simulink model "AWD_Test_VLC_ABS_Combined_FUZZY"  (Simulink 7.7)
settings: Solver=ode3  StartTime=0.0  StopTime=8  FixedStep=0.0001  RelTol=1e-3
undefined symbols (not defined in the file): Bx, By, Cx, Cy, Dx, Dy, Ex, Ey, g, GRR, GRR_E, hg, Jw, Jz, Lf, Lr, Lw, m, r0, Rw, rx1, rx2, ry1, ry2, T_Avail, Vx0, Vy0, wRL0
libraries: fuzblock x8, simulink x6
settings Model: Creator=ETLAB  LastModifiedBy=Kenny Schmutz
settings SolverCC: AlgebraicLoopSolver=LineSearch
settings DebuggingCC: InheritedTsInSrcMsg=none  FcnCallInpInsideContextMsg=Enable All

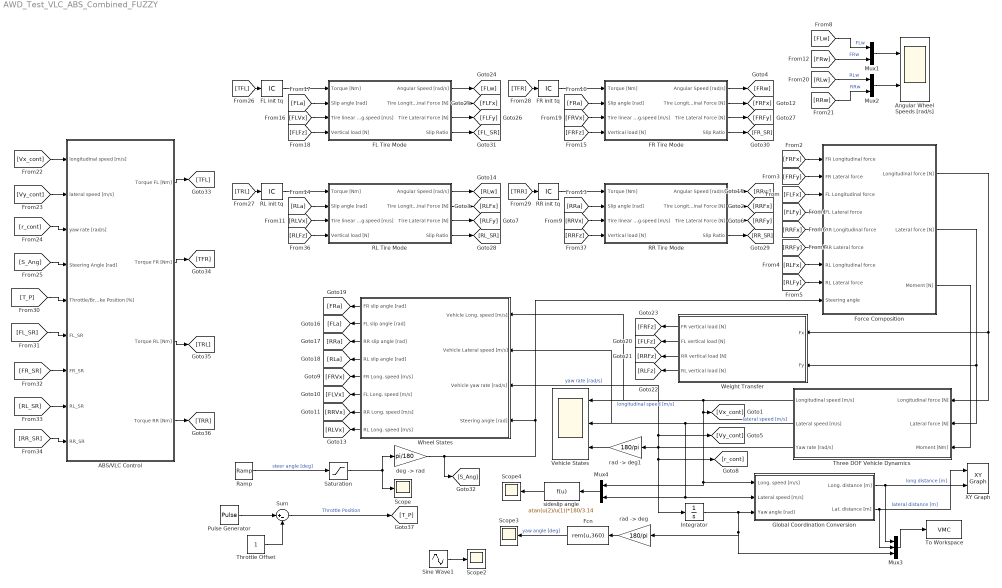
== system AWD_Test_VLC_ABS_Combined_FUZZY ==
  ABS/VLC Control : Subsystem
  Angular Wheel Speeds [rad/s] : Scope  NumInputPorts=2
      settings: YMin=-110~-110  YMax=30~30  SaveName=ScopeData7
  FL Tire Mode : Subsystem
      mask Display:
      | image(imread('Tire.bmp'),'center')
      | port_label('input', 1, 'Torque [Nm]')
      | port_label('input', 2, 'Slip angle [rad]')
      | port_label('input', 3, 'Long. speed [m/s]')
      | port_label('input', 4, 'Vertical load [N]')
      | port_label('output', 1, 'Angular speed [rad/s]')
      | port_label('output', 2, 'Long. force [N]')
      | port_label('output', 3, 'Lateral force [N]')
      | port_label('output', 4, 'Slip Ratio')
  FL init tq : InitialCondition  Value=0
  FR Tire Mode : Subsystem
      mask Display:
      | image(imread('Tire.bmp'),'center')
      | port_label('input', 1, 'Torque [Nm]')
      | port_label('input', 2, 'Slip angle [rad]')
      | port_label('input', 3, 'Long. speed [m/s]')
      | port_label('input', 4, 'Vertical load [N]')
      | port_label('output', 1, 'Angular speed [rad/s]')
      | port_label('output', 2, 'Long. force [N]')
      | port_label('output', 3, 'Lateral force [N]')
      | port_label('output', 4, 'Slip Ratio')
  FR init tq : InitialCondition  Value=0
  Fcn : Fcn  Expr=rem(u,360)
  Force Composition : Subsystem
  Global Coordination Conversion : Subsystem
  Integrator : Integrator
  Mux1 : Mux  Inputs=2
  Mux2 : Mux  Inputs=2
  Mux3 : Mux  Inputs=3
  Mux4 : Mux  Inputs=2
  Pulse Generator : DiscretePulseGenerator  PulseType=Time based  Amplitude=2  Period=8  PulseWidth=50
  RL Tire Mode : Subsystem
      mask Display:
      | image(imread('Tire.bmp'),'center')
      | port_label('input', 1, 'Torque [Nm]')
      | port_label('input', 2, 'Slip angle [rad]')
      | port_label('input', 3, 'Long. speed [m/s]')
      | port_label('input', 4, 'Vertical load [N]')
      | port_label('output', 1, 'Angular speed [rad/s]')
      | port_label('output', 2, 'Long. force [N]')
      | port_label('output', 3, 'Lateral force [N]')
      | port_label('output', 4, 'Slip Ratio')
  RL init tq : InitialCondition  Value=0
  RR Tire Mode : Subsystem
      mask Display:
      | image(imread('Tire.bmp'),'center')
      | port_label('input', 1, 'Torque [Nm]')
      | port_label('input', 2, 'Slip angle [rad]')
      | port_label('input', 3, 'Long. speed [m/s]')
      | port_label('input', 4, 'Vertical load [N]')
      | port_label('output', 1, 'Angular speed [rad/s]')
      | port_label('output', 2, 'Long. force [N]')
      | port_label('output', 3, 'Lateral force [N]')
      | port_label('output', 4, 'Slip Ratio')
  RR init tq : InitialCondition  Value=0
  Ramp : simulink/Sources/Ramp  SystemSampleTime=-1  slope=0  start=0  X0=0
  Saturation : Saturate  UpperLimit=10  LowerLimit=-10
  Scope{,2..4} (4 alike) : Scope
      Scope settings: YMin=0.93  YMax=1
      Scope2 settings: YMin=0.525  YMax=0.825  SaveName=ScopeData3
      Scope3 settings: SaveName=ScopeData5
      Scope4 settings: YMin=1.8e-014  YMax=2.5e-014  SaveName=ScopeData20
  Sine Wave1 : Sin  Frequency=0.5  SampleTime=0
  Sum : Sum  Inputs=|+-
  Three DOF Vehicle Dynamics : Subsystem
      mask Display:
      | image(imread('Vehicle.bmp'),'center')
      | port_label('input', 1, 'Longitudinal force [N]')
      | port_label('input', 2, 'Lateral force [N]')
      | port_label('input', 3, 'Moment [Nm]')
      | port_label('output', 1, 'Longitudinal speed [m/s]')
      | port_label('output', 2, 'Lateral speed [m/s]')
      | port_label('output', 3, 'Yaw rate [rad/s]')
  Throttle Offset : Constant
  To Workspace : ToWorkspace  VariableName=VMC  SampleTime=-1  SaveFormat=Array
  Vehicle States : Scope  NumInputPorts=3
      settings: TimeRange=6  YMin=2.5~-6e-018~-2.5e-016  YMax=35~5e-019~1.5e-015  SaveName=StatesOutpus1
  Weight Transfer : Subsystem
  Wheel States : Subsystem
  XY Graph : simulink/Sinks/XY Graph  SystemSampleTime=-1  xmin=-500  xmax=500  ymin=-500  ymax=500  st=-1
  "deg -> rad" : Gain  Gain=pi/180
  "rad -> deg" : Gain  Gain=180/pi
  "rad -> deg1" : Gain  Gain=180/pi
  sideslip angle : Fcn  Expr=atan(u(2)/u(1))*180/3.14
  wires:
  RL Tire Mode/2(Tire Longitudinal Force [N]) -> [RLFx]
  RL Tire Mode/1(Angular Speed [rad/s]) -> [RLw]
  [RLVx] -> RL Tire Mode/3(Tire linear Long.speed [m/s])
  Wheel States/5(FR Long. speed [m/s]) -> [FRVx]
  Wheel States/6(FL Long. speed [m/s]) -> [FLVx]
  Wheel States/7(RR Long. speed [m/s]) -> [RRVx]
  Wheel States/8(RL Long. speed [m/s]) -> [RLVx]
  Three DOF Vehicle Dynamics/3(Yaw rate [rad/s]) -> "rad -> deg1"/1, Wheel States/3(Vehicle yaw rate [rad/s]), [Vy_cont], Integrator/1, [r_cont]  "yaw rate [rad/s]"
  Three DOF Vehicle Dynamics/2(Lateral speed [m/s]) -> Wheel States/2(Vehicle Lateral speed [m/s]), Global Coordination Conversion/2(Lateral speed [m/s]), Mux4/2, Vehicle States/2  "lateral speed [m/s]"
  Three DOF Vehicle Dynamics/1(Longitudinal speed [m/s]) -> Wheel States/1(Vehicle Long. speed [m/s]), Vehicle States/1, Global Coordination Conversion/1(Long. speed [m/s]), Mux4/1, [Vx_cont]  "longitudinal speed [m/s]"
  Wheel States/1("FR slip angle [rad] ") -> [FRa]
  Wheel States/2("FL slip angle [rad] ") -> [FLa]
  Wheel States/3("RR slip angle [rad] ") -> [RRa]
  Wheel States/4("RL slip angle [rad] ") -> [RLa]
  [RLa] -> RL Tire Mode/2(Slip angle [rad])
  Force Composition/1(Longitudinal force [N]) -> Weight Transfer/1(Fx), Three DOF Vehicle Dynamics/1(Longitudinal force [N])
  [FRFx] -> Force Composition/1(FR Longitudinal force)
  [FRFy] -> Force Composition/2(FR Lateral force)
  [FLFx] -> Force Composition/3(FL Longitudinal force)
  [FLFy] -> Force Composition/4(FL Lateral force)
  [RRFx] -> Force Composition/5(RR Longitudinal force)
  [RRFy] -> Force Composition/6(RR Lateral force)
  [RLFx] -> Force Composition/7(RL Longitudinal force)
  [RLFy] -> Force Composition/8(RL Lateral force)
  "deg -> rad"/1 -> Wheel States/4(Steering angle [rad]), Force Composition/9(Steering angle), [S_Ang]
  "rad -> deg"/1 -> Fcn/1
  Fcn/1 -> Scope3/1  "yaw angle [deg]"
  Global Coordination Conversion/1(Long. distance [m]) -> XY Graph/2, Mux3/1  "long distance [m]"
  Global Coordination Conversion/2(Lat. distance [m]) -> XY Graph/1, Mux3/2  "lateral distance [m]"
  Weight Transfer/1(FR vertical load [N]) -> [FRFz]
  Weight Transfer/2(FL vertical load [N]) -> [FLFz]
  Weight Transfer/3(RR vertical load [N]) -> [RRFz]
  Weight Transfer/4(RL vertical load [N]) -> [RLFz]
  [RLFz] -> RL Tire Mode/4(Vertical load [N])
  Force Composition/2(Lateral force [N]) -> Weight Transfer/2(Fy), Three DOF Vehicle Dynamics/2(Lateral force [N])
  Integrator/1 -> Global Coordination Conversion/3(Yaw angle [rad]), "rad -> deg"/1, Mux3/3
  RL Tire Mode/3(Tire Lateral Force [N]) -> [RLFy]
  [RRa] -> RR Tire Mode/2(Slip angle [rad])
  [RRVx] -> RR Tire Mode/3(Tire linear Long.speed [m/s])
  [RRFz] -> RR Tire Mode/4(Vertical load [N])
  RR Tire Mode/1(Angular Speed [rad/s]) -> [RRw]
  RR Tire Mode/2(Tire Longitudinal Force [N]) -> [RRFx]
  RR Tire Mode/3(Tire Lateral Force [N]) -> [RRFy]
  Force Composition/3(Moment [N]) -> Three DOF Vehicle Dynamics/3(Moment [Nm])
  "rad -> deg1"/1 -> Vehicle States/3
  Mux4/1 -> sideslip angle/1
  sideslip angle/1 -> Scope4/1
  Ramp/1 -> Saturation/1  "steer angle [deg]"
  Sine Wave1/1 -> Scope2/1
  FL Tire Mode/2(Tire Longitudinal Force [N]) -> [FLFx]
  FL Tire Mode/1(Angular Speed [rad/s]) -> [FLw]
  [FLVx] -> FL Tire Mode/3(Tire linear Long.speed [m/s])
  FL init tq/1 -> FL Tire Mode/1(Torque [Nm])
  [FLa] -> FL Tire Mode/2(Slip angle [rad])
  [FLFz] -> FL Tire Mode/4(Vertical load [N])
  FL Tire Mode/3(Tire Lateral Force [N]) -> [FLFy]
  [FRa] -> FR Tire Mode/2(Slip angle [rad])
  [FRVx] -> FR Tire Mode/3(Tire linear Long.speed [m/s])
  [FRFz] -> FR Tire Mode/4(Vertical load [N])
  FR Tire Mode/1(Angular Speed [rad/s]) -> [FRw]
  FR Tire Mode/2(Tire Longitudinal Force [N]) -> [FRFx]
  FR Tire Mode/3(Tire Lateral Force [N]) -> [FRFy]
  Saturation/1 -> "deg -> rad"/1, Scope/1
  [FLw] -> Mux1/1  "FLw"
  [FRw] -> Mux1/2  "FRw"
  [RLw] -> Mux2/1  "RLw"
  [RRw] -> Mux2/2  "RRw"
  Mux1/1 -> Angular Wheel Speeds [rad/s]/1
  Mux2/1 -> Angular Wheel Speeds [rad/s]/2
  [Vx_cont] -> ABS/VLC Control/1(longitudinal speed [m/s])
  [Vy_cont] -> ABS/VLC Control/2(lateral speed [m/s])
  [r_cont] -> ABS/VLC Control/3(yaw rate [rad/s])
  RL Tire Mode/4("Slip Ratio ") -> [RL_SR]
  RR Tire Mode/4(Slip Ratio) -> [RR_SR]
  FR Tire Mode/4(Slip Ratio) -> [FR_SR]
  FL Tire Mode/4(Slip Ratio) -> [FL_SR]
  [S_Ang] -> ABS/VLC Control/4(Steering Angle [rad])
  [TFL] -> FL init tq/1
  RL init tq/1 -> RL Tire Mode/1(Torque [Nm])
  [TRL] -> RL init tq/1
  FR init tq/1 -> FR Tire Mode/1(Torque [Nm])
  [TFR] -> FR init tq/1
  RR init tq/1 -> RR Tire Mode/1(Torque [Nm])
  [TRR] -> RR init tq/1
  Sum/1 -> [T_P]  "Throttle Position"
  [T_P] -> ABS/VLC Control/5(Throttle/Brake Position [%])
  [FL_SR] -> ABS/VLC Control/6(FL_SR)
  [FR_SR] -> ABS/VLC Control/7(FR_SR)
  [RL_SR] -> ABS/VLC Control/8(RL_SR)
  [RR_SR] -> ABS/VLC Control/9(RR_SR)
  ABS/VLC Control/1(Torque FL [Nm]) -> [TFL]
  ABS/VLC Control/2(Torque FR [Nm]) -> [TFR]
  ABS/VLC Control/3(Torque RL [Nm]) -> [TRL]
  ABS/VLC Control/4(Torque RR [Nm]) -> [TRR]
  Mux3/1 -> To Workspace/1
  Pulse Generator/1 -> Sum/1
  Throttle Offset/1 -> Sum/2

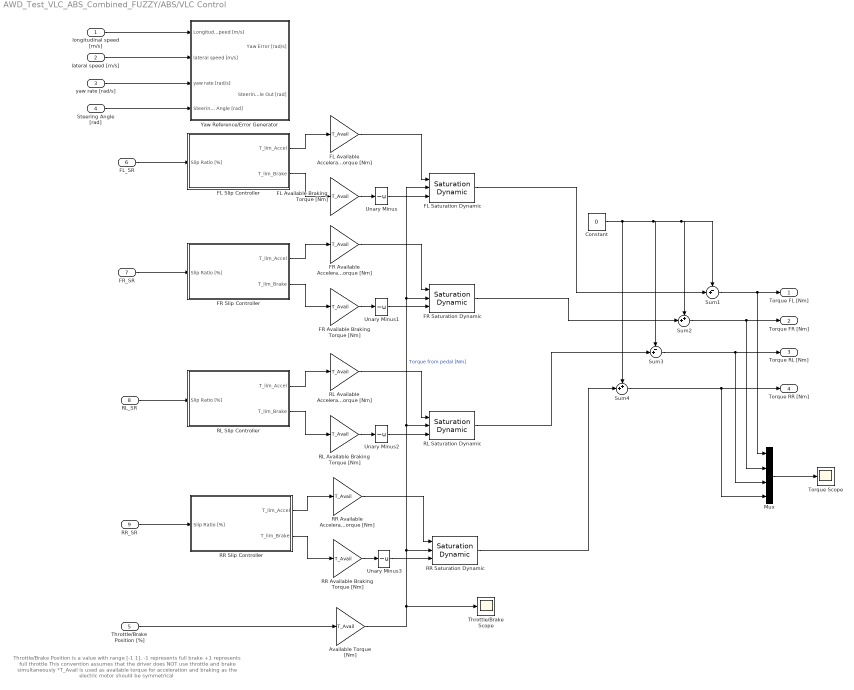
== system AWD_Test_VLC_ABS_Combined_FUZZY/ABS/VLC Control ==
  note: Throttle/Brake Position is a value with range [-1 1].
      | -1 represents full brake
      | +1 represents full throttle
      | This convention assumes that the driver does NOT use throttle and brake simultaneously
      |
      | *T_Avail is used as available torque for acceleration and braking as the electric motor should be symmetrical
  longitudinal speed [m/s] : Inport
  lateral speed [m/s] : Inport  Port=2
  yaw rate [rad/s] : Inport  Port=3
  Steering Angle [rad] : Inport  Port=4
  Throttle/Brake Position [%] : Inport  Port=5
  FL_SR : Inport  Port=6
  FR_SR : Inport  Port=7
  RL_SR : Inport  Port=8
  RR_SR : Inport  Port=9
  Available Torque [Nm] : Gain  Gain=T_Avail
  Constant : Constant  Value=0
  FL Available Acceleration Torque [Nm] : Gain  Gain=T_Avail
  FL Available Braking Torque [Nm] : Gain  Gain=T_Avail
  FL Saturation Dynamic : simulink/Discontinuities/Saturation Dynamic  SystemSampleTime=-1  OutMin=[]  OutMax=[]  OutDataTypeStr=Inherit: Same as second input  OutDataType=fixdt(1, 16)  OutScaling=2^-10  DoSatur=off
  FL Slip Controller : Subsystem
  FR Available Acceleration Torque [Nm] : Gain  Gain=T_Avail
  FR Available Braking Torque [Nm] : Gain  Gain=T_Avail
  FR Saturation Dynamic : simulink/Discontinuities/Saturation Dynamic  SystemSampleTime=-1  OutMin=[]  OutMax=[]  OutDataTypeStr=Inherit: Same as second input  OutDataType=fixdt(1, 16)  OutScaling=2^-10  DoSatur=off
  FR Slip Controller : Subsystem
  Mux : Mux
  RL Available Acceleration Torque [Nm] : Gain  Gain=T_Avail
  RL Available Braking Torque [Nm] : Gain  Gain=T_Avail
  RL Saturation Dynamic : simulink/Discontinuities/Saturation Dynamic  SystemSampleTime=-1  OutMin=[]  OutMax=[]  OutDataTypeStr=Inherit: Same as second input  OutDataType=fixdt(1, 16)  OutScaling=2^-10  DoSatur=off
  RL Slip Controller : Subsystem
  RR Available Acceleration Torque [Nm] : Gain  Gain=T_Avail
  RR Available Braking Torque [Nm] : Gain  Gain=T_Avail
  RR Saturation Dynamic : simulink/Discontinuities/Saturation Dynamic  SystemSampleTime=-1  OutMin=[]  OutMax=[]  OutDataTypeStr=Inherit: Same as second input  OutDataType=fixdt(1, 16)  OutScaling=2^-10  DoSatur=off
  RR Slip Controller : Subsystem
  Sum1 : Sum  Inputs=-+|
  Sum2 : Sum  Inputs=++|
  Sum3 : Sum  Inputs=-+|
  Sum4 : Sum  Inputs=++|
  Throttle/Brake Scope : Scope
      settings: YMin=150  YMax=150  SaveName=ScopeData9
  Torque Scope : Scope
      settings: YMin=-150  YMax=0  SaveName=ScopeData16
  Unary Minus{,1..3} (4 alike) : UnaryMinus
  Yaw Reference/Error Generator : Subsystem
  Torque FL [Nm] : Outport
  Torque FR [Nm] : Outport  Port=2
  Torque RL [Nm] : Outport  Port=3
  Torque RR [Nm] : Outport  Port=4
  wires:
  Sum1/1 -> Torque FL [Nm]/1, Mux/1
  Sum2/1 -> Torque FR [Nm]/1, Mux/2
  Sum3/1 -> Torque RL [Nm]/1, Mux/3
  Sum4/1 -> Torque RR [Nm]/1, Mux/4
  Throttle/Brake Position [%]/1 -> Available Torque [Nm]/1
  Available Torque [Nm]/1 -> RR Saturation Dynamic/2, RL Saturation Dynamic/2, FR Saturation Dynamic/2, FL Saturation Dynamic/2, Throttle/Brake Scope/1  "Torque from pedal [Nm]"
  FL_SR/1 -> FL Slip Controller/1(Slip Ratio [%])
  FL Slip Controller/1(T_lim_Accel) -> FL Available Acceleration Torque [Nm]/1
  FL Available Acceleration Torque [Nm]/1 -> FL Saturation Dynamic/1
  Unary Minus/1 -> FL Saturation Dynamic/3
  FL Saturation Dynamic/1 -> Sum1/2
  Constant/1 -> Sum4/1, Sum3/1, Sum1/1, Sum2/1
  Mux/1 -> Torque Scope/1
  FL Slip Controller/2(T_lim_Brake) -> FL Available Braking Torque [Nm]/1
  FL Available Braking Torque [Nm]/1 -> Unary Minus/1
  FR_SR/1 -> FR Slip Controller/1(Slip Ratio [%])
  FR Slip Controller/1(T_lim_Accel) -> FR Available Acceleration Torque [Nm]/1
  FR Available Acceleration Torque [Nm]/1 -> FR Saturation Dynamic/1
  Unary Minus1/1 -> FR Saturation Dynamic/3
  FR Slip Controller/2(T_lim_Brake) -> FR Available Braking Torque [Nm]/1
  FR Available Braking Torque [Nm]/1 -> Unary Minus1/1
  RL_SR/1 -> RL Slip Controller/1(Slip Ratio [%])
  RL Slip Controller/1(T_lim_Accel) -> RL Available Acceleration Torque [Nm]/1
  RL Available Acceleration Torque [Nm]/1 -> RL Saturation Dynamic/1
  Unary Minus2/1 -> RL Saturation Dynamic/3
  RL Slip Controller/2(T_lim_Brake) -> RL Available Braking Torque [Nm]/1
  RL Available Braking Torque [Nm]/1 -> Unary Minus2/1
  RR Slip Controller/1(T_lim_Accel) -> RR Available Acceleration Torque [Nm]/1
  RR Available Acceleration Torque [Nm]/1 -> RR Saturation Dynamic/1
  Unary Minus3/1 -> RR Saturation Dynamic/3
  RR Slip Controller/2(T_lim_Brake) -> RR Available Braking Torque [Nm]/1
  RR Available Braking Torque [Nm]/1 -> Unary Minus3/1
  RR_SR/1 -> RR Slip Controller/1(Slip Ratio [%])
  FR Saturation Dynamic/1 -> Sum2/2
  RL Saturation Dynamic/1 -> Sum3/2
  RR Saturation Dynamic/1 -> Sum4/2
  longitudinal speed [m/s]/1 -> Yaw Reference/Error Generator/1(Longitudinal Speed [m/s])
  lateral speed [m/s]/1 -> Yaw Reference/Error Generator/2(lateral speed [m/s])
  yaw rate [rad/s]/1 -> Yaw Reference/Error Generator/3(yaw rate [rad/s])
  Steering Angle [rad]/1 -> Yaw Reference/Error Generator/4(Steering Angle [rad])

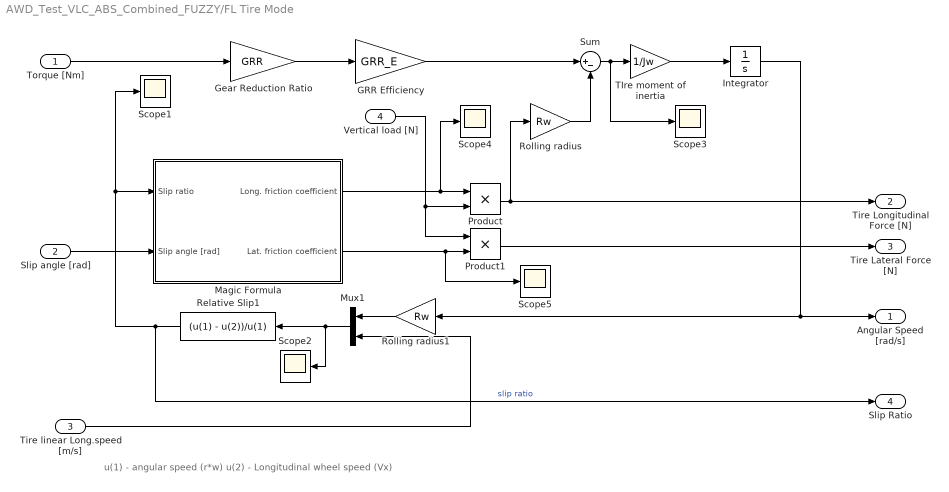
== system AWD_Test_VLC_ABS_Combined_FUZZY/FL Tire Mode ==
  note: u(1) - angular speed (r*w)
      | u(2) - Longitudinal wheel speed (Vx)
  Torque [Nm] : Inport
  Slip angle [rad] : Inport  Port=2
  Tire linear Long.speed [m/s] : Inport  Port=3
  Vertical load [N] : Inport  Port=4
  GRR Efficiency : Gain  Gain=GRR_E  SaturateOnIntegerOverflow=on  OutDataTypeStr=Inherit: Same as input  ParamDataTypeStr=Inherit: Same as input
  Gear Reduction Ratio : Gain  Gain=GRR  SaturateOnIntegerOverflow=on  OutDataTypeStr=Inherit: Same as input  ParamDataTypeStr=Inherit: Same as input
  Integrator : Integrator  InitialCondition=wRL0
  Magic Formula : Subsystem
      mask Type: Magic Formula (Combined Slip)
      mask Display:
      | image(imread('Magic formula.jpg'),'center')
      | port_label('input', 1, 'slip ratio')
      | port_label('input', 2, 'slip angle')
      | port_label('output', 1, 'Mux')
      | port_label('output', 2, 'Muy')
  Mux1 : Mux  Inputs=2
  Product : Product  RndMeth=Zero
  Product1 : Product  RndMeth=Zero
  Relative Slip1 : Fcn  Expr=(u(1) - u(2))/u(1)
  Rolling radius : Gain  Gain=Rw  SaturateOnIntegerOverflow=on  OutDataTypeStr=Inherit: Same as input  ParamDataTypeStr=Inherit: Same as input
  Rolling radius1 : Gain  Gain=Rw  SaturateOnIntegerOverflow=on  OutDataTypeStr=Inherit: Same as input  ParamDataTypeStr=Inherit: Same as input
  Scope{1..5} (5 alike) : Scope
      Scope1 settings: YMin=0.122  YMax=0.122004  SaveName=ScopeData2
      Scope2 settings: TimeRange=6  YMin=44  YMax=50.5  SaveName=ScopeData11
      Scope3 settings: YMin=5.45315  YMax=5.45315  SaveName=ScopeData14
      Scope4 settings: YMin=0.775111  YMax=0.856701  SaveName=ScopeData13
      Scope5 settings: YMin=-0.14725  YMax=-0.1463  SaveName=ScopeData15
  Sum : Sum  Inputs=|+-
  TIre moment of inertia : Gain  Gain=1/Jw  SaturateOnIntegerOverflow=on  OutDataTypeStr=Inherit: Same as input  ParamDataTypeStr=Inherit: Same as input
  Angular Speed [rad/s] : Outport
  Tire Longitudinal Force [N] : Outport  Port=2
  Tire Lateral Force [N] : Outport  Port=3
  Slip Ratio : Outport  Port=4
  wires:
  Slip angle [rad]/1 -> Magic Formula/2(Slip angle [rad])
  Relative Slip1/1 -> Magic Formula/1(Slip ratio), Scope1/1, Slip Ratio/1  "slip ratio"
  Tire linear Long.speed [m/s]/1 -> Mux1/2
  Torque [Nm]/1 -> Gear Reduction Ratio/1
  Sum/1 -> TIre moment of inertia/1, Scope3/1
  TIre moment of inertia/1 -> Integrator/1
  Integrator/1 -> Angular Speed [rad/s]/1, Rolling radius1/1
  Rolling radius/1 -> Sum/2
  Mux1/1 -> Relative Slip1/1, Scope2/1
  Rolling radius1/1 -> Mux1/1
  Magic Formula/1(Long. friction coefficient) -> Product/1, Scope4/1
  Magic Formula/2(Lat. friction coefficient) -> Product1/2, Scope5/1
  Product/1 -> Rolling radius/1, Tire Longitudinal Force [N]/1
  Vertical load [N]/1 -> Product/2, Product1/1
  Product1/1 -> Tire Lateral Force [N]/1
  Gear Reduction Ratio/1 -> GRR Efficiency/1
  GRR Efficiency/1 -> Sum/1

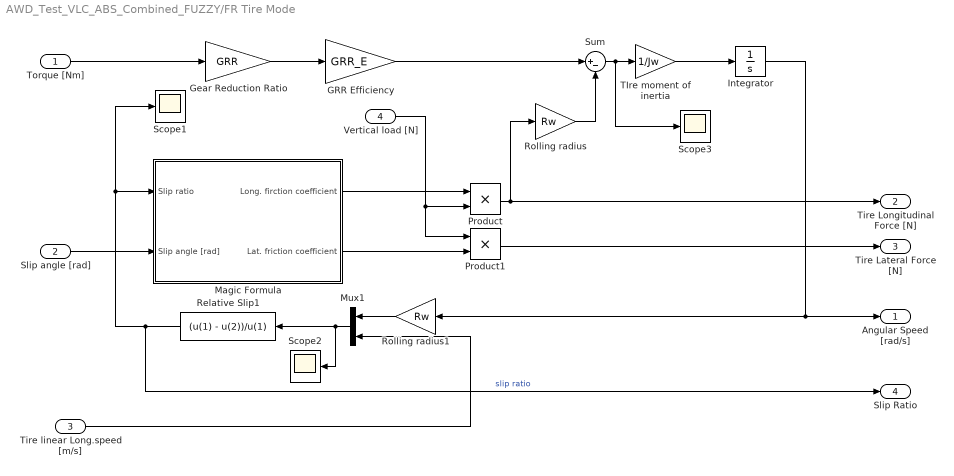
== system AWD_Test_VLC_ABS_Combined_FUZZY/FR Tire Mode ==
  Torque [Nm] : Inport
  Slip angle [rad] : Inport  Port=2
  Tire linear Long.speed [m/s] : Inport  Port=3
  Vertical load [N] : Inport  Port=4
  GRR Efficiency : Gain  Gain=GRR_E  SaturateOnIntegerOverflow=on  OutDataTypeStr=Inherit: Same as input  ParamDataTypeStr=Inherit: Same as input
  Gear Reduction Ratio : Gain  Gain=GRR  SaturateOnIntegerOverflow=on  OutDataTypeStr=Inherit: Same as input  ParamDataTypeStr=Inherit: Same as input
  Integrator : Integrator  InitialCondition=wRL0
  Magic Formula : Subsystem
      mask Type: Magic Formula (Combined Slip)
      mask Display:
      | image(imread('Magic formula.jpg'),'center')
      | port_label('input', 1, 'slip ratio')
      | port_label('input', 2, 'slip angle')
      | port_label('output', 1, 'Mux')
      | port_label('output', 2, 'Muy')
  Mux1 : Mux  Inputs=2
  Product : Product  RndMeth=Zero
  Product1 : Product  RndMeth=Zero
  Relative Slip1 : Fcn  Expr=(u(1) - u(2))/u(1)
  Rolling radius : Gain  Gain=Rw  SaturateOnIntegerOverflow=on  OutDataTypeStr=Inherit: Same as input  ParamDataTypeStr=Inherit: Same as input
  Rolling radius1 : Gain  Gain=Rw  SaturateOnIntegerOverflow=on  OutDataTypeStr=Inherit: Same as input  ParamDataTypeStr=Inherit: Same as input
  Scope1 : Scope
      settings: YMin=0.0014905  YMax=0.0014955  SaveName=ScopeData2
  Scope2 : Scope
      settings: YMin=0.001  YMax=0.013  SaveName=ScopeData11
  Scope3 : Scope
      settings: SaveName=ScopeData14
  Sum : Sum  Inputs=|+-
  TIre moment of inertia : Gain  Gain=1/Jw  SaturateOnIntegerOverflow=on  OutDataTypeStr=Inherit: Same as input  ParamDataTypeStr=Inherit: Same as input
  Angular Speed [rad/s] : Outport
  Tire Longitudinal Force [N] : Outport  Port=2
  Tire Lateral Force [N] : Outport  Port=3
  Slip Ratio : Outport  Port=4
  wires:
  Product1/1 -> Tire Lateral Force [N]/1
  Vertical load [N]/1 -> Product1/1, Product/2
  Product/1 -> Tire Longitudinal Force [N]/1, Rolling radius/1
  Magic Formula/2(Lat. friction coefficient) -> Product1/2
  Magic Formula/1(Long. firction coefficient) -> Product/1
  Rolling radius1/1 -> Mux1/1
  Mux1/1 -> Relative Slip1/1, Scope2/1
  Rolling radius/1 -> Sum/2
  Integrator/1 -> Rolling radius1/1, Angular Speed [rad/s]/1
  TIre moment of inertia/1 -> Integrator/1
  Sum/1 -> Scope3/1, TIre moment of inertia/1
  Torque [Nm]/1 -> Gear Reduction Ratio/1
  Tire linear Long.speed [m/s]/1 -> Mux1/2
  Relative Slip1/1 -> Scope1/1, Magic Formula/1(Slip ratio), Slip Ratio/1  "slip ratio"
  Slip angle [rad]/1 -> Magic Formula/2(Slip angle [rad])
  Gear Reduction Ratio/1 -> GRR Efficiency/1
  GRR Efficiency/1 -> Sum/1

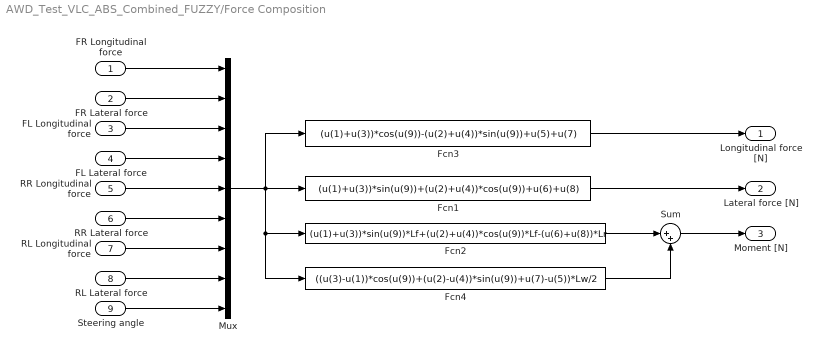
== system AWD_Test_VLC_ABS_Combined_FUZZY/Force Composition ==
  FR Longitudinal force : Inport
  FR Lateral force : Inport  Port=2
  FL Longitudinal force : Inport  Port=3
  FL Lateral force : Inport  Port=4
  RR Longitudinal force : Inport  Port=5
  RR Lateral force : Inport  Port=6
  RL Longitudinal force : Inport  Port=7
  RL Lateral force : Inport  Port=8
  Steering angle : Inport  Port=9
  Fcn1 : Fcn  Expr=(u(1)+u(3))*sin(u(9))+(u(2)+u(4))*cos(u(9))+u(6)+u(8)
  Fcn2 : Fcn  Expr=(u(1)+u(3))*sin(u(9))*Lf+(u(2)+u(4))*cos(u(9))*Lf-(u(6)+u(8))*Lr
  Fcn3 : Fcn  Expr=(u(1)+u(3))*cos(u(9))-(u(2)+u(4))*sin(u(9))+u(5)+u(7)
  Fcn4 : Fcn  Expr=((u(3)-u(1))*cos(u(9))+(u(2)-u(4))*sin(u(9))+u(7)-u(5))*Lw/2
  Mux : Mux  Inputs=9
  Sum : Sum  Inputs=|++
  Longitudinal force [N] : Outport
  Lateral force [N] : Outport  Port=2
  Moment [N] : Outport  Port=3
  wires:
  Mux/1 -> Fcn3/1, Fcn1/1, Fcn2/1, Fcn4/1
  Fcn3/1 -> Longitudinal force [N]/1
  Fcn1/1 -> Lateral force [N]/1
  Sum/1 -> Moment [N]/1
  Fcn2/1 -> Sum/1
  Fcn4/1 -> Sum/2
  FR Longitudinal force/1 -> Mux/1
  FR Lateral force/1 -> Mux/2
  FL Longitudinal force/1 -> Mux/3
  FL Lateral force/1 -> Mux/4
  RR Longitudinal force/1 -> Mux/5
  RR Lateral force/1 -> Mux/6
  RL Longitudinal force/1 -> Mux/7
  RL Lateral force/1 -> Mux/8
  Steering angle/1 -> Mux/9

== system AWD_Test_VLC_ABS_Combined_FUZZY/Global Coordination Conversion ==
  Long. speed [m/s] : Inport
  Lateral speed [m/s] : Inport  Port=2
  Yaw angle [rad] : Inport  Port=3
  Fcn : Fcn  Expr=cos(u(3))*u(1)-sin(u(3))*u(2)
  Fcn1 : Fcn  Expr=sin(u(3))*u(1)+cos(u(3))*u(2)
  Integrator : Integrator
  Integrator1 : Integrator
  Mux : Mux  Inputs=3
  Long. distance [m] : Outport
  Lat. distance [m] : Outport  Port=2
  wires:
  Long. speed [m/s]/1 -> Mux/1
  Lateral speed [m/s]/1 -> Mux/2
  Yaw angle [rad]/1 -> Mux/3
  Mux/1 -> Fcn/1, Fcn1/1
  Fcn/1 -> Integrator/1
  Fcn1/1 -> Integrator1/1
  Integrator/1 -> Long. distance [m]/1
  Integrator1/1 -> Lat. distance [m]/1

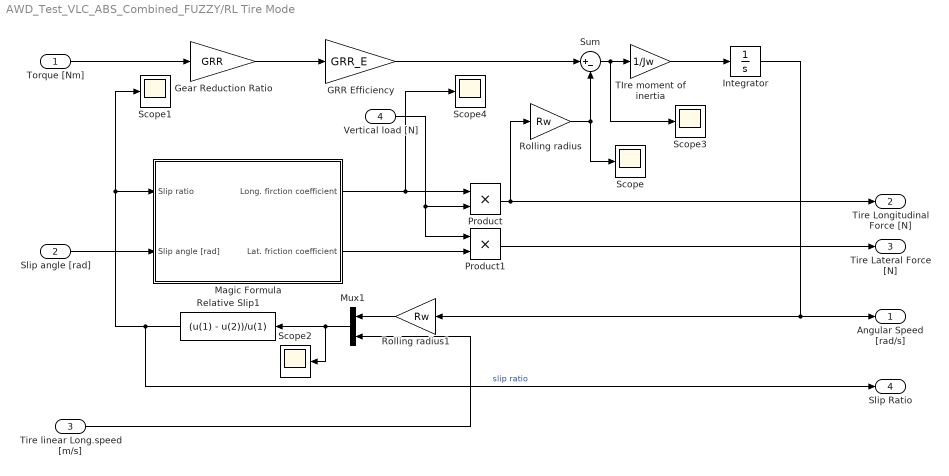
== system AWD_Test_VLC_ABS_Combined_FUZZY/RL Tire Mode ==
  Torque [Nm] : Inport
  Slip angle [rad] : Inport  Port=2
  Tire linear Long.speed [m/s] : Inport  Port=3
  Vertical load [N] : Inport  Port=4
  GRR Efficiency : Gain  Gain=GRR_E  SaturateOnIntegerOverflow=on  OutDataTypeStr=Inherit: Same as input  ParamDataTypeStr=Inherit: Same as input
  Gear Reduction Ratio : Gain  Gain=GRR  SaturateOnIntegerOverflow=on  OutDataTypeStr=Inherit: Same as input  ParamDataTypeStr=Inherit: Same as input
  Integrator : Integrator  InitialCondition=wRL0
  Magic Formula : Subsystem
      mask Type: Magic Formula (Combined Slip)
      mask Display:
      | image(imread('Magic formula.jpg'),'center')
      | port_label('input', 1, 'slip ratio')
      | port_label('input', 2, 'slip angle')
      | port_label('output', 1, 'Mux')
      | port_label('output', 2, 'Muy')
  Mux1 : Mux  Inputs=2
  Product : Product  RndMeth=Zero
  Product1 : Product  RndMeth=Zero
  Relative Slip1 : Fcn  Expr=(u(1) - u(2))/u(1)
  Rolling radius : Gain  Gain=Rw  SaturateOnIntegerOverflow=on  OutDataTypeStr=Inherit: Same as input  ParamDataTypeStr=Inherit: Same as input
  Rolling radius1 : Gain  Gain=Rw  SaturateOnIntegerOverflow=on  OutDataTypeStr=Inherit: Same as input  ParamDataTypeStr=Inherit: Same as input
  Scope{,1..4} (5 alike) : Scope
      Scope settings: SaveName=ScopeData10
      Scope1 settings: YMin=0.0014905  YMax=0.0014955  SaveName=ScopeData2
      Scope2 settings: YMin=0.001  YMax=0.013  SaveName=ScopeData11
      Scope3 settings: SaveName=ScopeData14
      Scope4 settings: YMin=-0.8  YMax=0.8  SaveName=ScopeData12
  Sum : Sum  Inputs=|+-
  TIre moment of inertia : Gain  Gain=1/Jw  SaturateOnIntegerOverflow=on  OutDataTypeStr=Inherit: Same as input  ParamDataTypeStr=Inherit: Same as input
  Angular Speed [rad/s] : Outport
  Tire Longitudinal Force [N] : Outport  Port=2
  Tire Lateral Force [N] : Outport  Port=3
  "Slip Ratio " : Outport  Port=4
  wires:
  Slip angle [rad]/1 -> Magic Formula/2(Slip angle [rad])
  Relative Slip1/1 -> Magic Formula/1(Slip ratio), Scope1/1, "Slip Ratio "/1  "slip ratio"
  Tire linear Long.speed [m/s]/1 -> Mux1/2
  Torque [Nm]/1 -> Gear Reduction Ratio/1
  Sum/1 -> TIre moment of inertia/1, Scope3/1
  TIre moment of inertia/1 -> Integrator/1
  Integrator/1 -> Angular Speed [rad/s]/1, Rolling radius1/1
  Rolling radius/1 -> Sum/2, Scope/1
  Mux1/1 -> Relative Slip1/1, Scope2/1
  Rolling radius1/1 -> Mux1/1
  Magic Formula/1(Long. firction coefficient) -> Product/1, Scope4/1
  Magic Formula/2(Lat. friction coefficient) -> Product1/2
  Product/1 -> Rolling radius/1, Tire Longitudinal Force [N]/1
  Vertical load [N]/1 -> Product/2, Product1/1
  Product1/1 -> Tire Lateral Force [N]/1
  Gear Reduction Ratio/1 -> GRR Efficiency/1
  GRR Efficiency/1 -> Sum/1

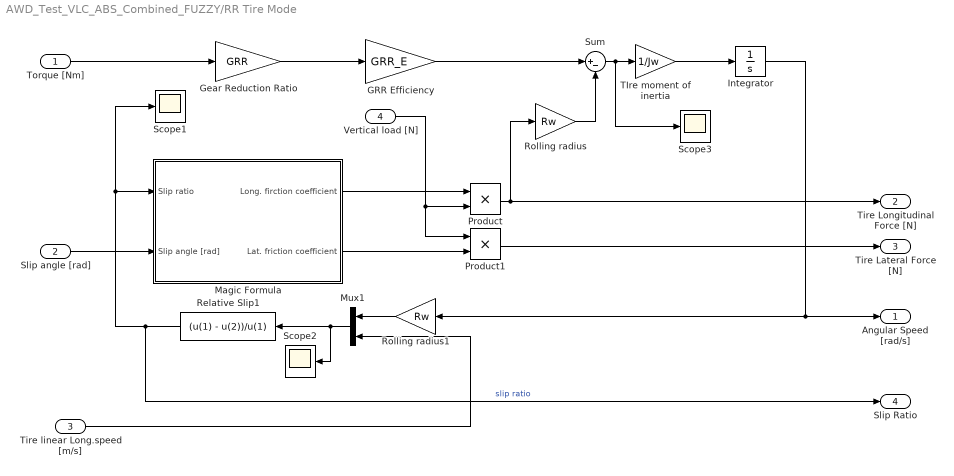
== system AWD_Test_VLC_ABS_Combined_FUZZY/RR Tire Mode ==
  Torque [Nm] : Inport
  Slip angle [rad] : Inport  Port=2
  Tire linear Long.speed [m/s] : Inport  Port=3
  Vertical load [N] : Inport  Port=4
  GRR Efficiency : Gain  Gain=GRR_E  SaturateOnIntegerOverflow=on  OutDataTypeStr=Inherit: Same as input  ParamDataTypeStr=Inherit: Same as input
  Gear Reduction Ratio : Gain  Gain=GRR  SaturateOnIntegerOverflow=on  OutDataTypeStr=Inherit: Same as input  ParamDataTypeStr=Inherit: Same as input
  Integrator : Integrator  InitialCondition=wRL0
  Magic Formula : Subsystem
      mask Type: Magic Formula (Combined Slip)
      mask Display:
      | image(imread('Magic formula.jpg'),'center')
      | port_label('input', 1, 'slip ratio')
      | port_label('input', 2, 'slip angle')
      | port_label('output', 1, 'Mux')
      | port_label('output', 2, 'Muy')
  Mux1 : Mux  Inputs=2
  Product : Product  RndMeth=Zero
  Product1 : Product  RndMeth=Zero
  Relative Slip1 : Fcn  Expr=(u(1) - u(2))/u(1)
  Rolling radius : Gain  Gain=Rw  SaturateOnIntegerOverflow=on  OutDataTypeStr=Inherit: Same as input  ParamDataTypeStr=Inherit: Same as input
  Rolling radius1 : Gain  Gain=Rw  SaturateOnIntegerOverflow=on  OutDataTypeStr=Inherit: Same as input  ParamDataTypeStr=Inherit: Same as input
  Scope1 : Scope
      settings: YMin=0.0014905  YMax=0.0014955  SaveName=ScopeData2
  Scope2 : Scope
      settings: YMin=38.75  YMax=40.75  SaveName=ScopeData11
  Scope3 : Scope
      settings: YMin=709.756  YMax=709.758  SaveName=ScopeData14
  Sum : Sum  Inputs=|+-
  TIre moment of inertia : Gain  Gain=1/Jw  SaturateOnIntegerOverflow=on  OutDataTypeStr=Inherit: Same as input  ParamDataTypeStr=Inherit: Same as input
  Angular Speed [rad/s] : Outport
  Tire Longitudinal Force [N] : Outport  Port=2
  Tire Lateral Force [N] : Outport  Port=3
  Slip Ratio : Outport  Port=4
  wires:
  Product1/1 -> Tire Lateral Force [N]/1
  Vertical load [N]/1 -> Product1/1, Product/2
  Product/1 -> Tire Longitudinal Force [N]/1, Rolling radius/1
  Magic Formula/2(Lat. friction coefficient) -> Product1/2
  Magic Formula/1(Long. firction coefficient) -> Product/1
  Rolling radius1/1 -> Mux1/1
  Mux1/1 -> Relative Slip1/1, Scope2/1
  Rolling radius/1 -> Sum/2
  Integrator/1 -> Rolling radius1/1, Angular Speed [rad/s]/1
  TIre moment of inertia/1 -> Integrator/1
  Sum/1 -> Scope3/1, TIre moment of inertia/1
  Torque [Nm]/1 -> Gear Reduction Ratio/1
  Tire linear Long.speed [m/s]/1 -> Mux1/2
  Relative Slip1/1 -> Scope1/1, Magic Formula/1(Slip ratio), Slip Ratio/1  "slip ratio"
  Slip angle [rad]/1 -> Magic Formula/2(Slip angle [rad])
  Gear Reduction Ratio/1 -> GRR Efficiency/1
  GRR Efficiency/1 -> Sum/1

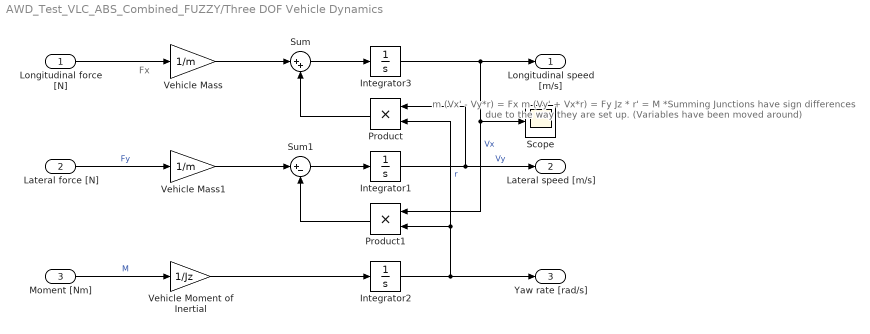
== system AWD_Test_VLC_ABS_Combined_FUZZY/Three DOF Vehicle Dynamics ==
  note: m (Vx' - Vy*r) = Fx
      | m (Vy' + Vx*r) = Fy
      |
      | Jz * r' = M
      |
      | *Summing Junctions have sign differences due to
      | the way they are set up. (Variables have been moved around)
  note: Fx
  Longitudinal force [N] : Inport
  Lateral force [N] : Inport  Port=2
  Moment [Nm] : Inport  Port=3
  Integrator1 : Integrator  InitialCondition=Vy0  UpperSaturationLimit=1000  LowerSaturationLimit=0
  Integrator2 : Integrator  InitialCondition=r0
  Integrator3 : Integrator  InitialCondition=Vx0  UpperSaturationLimit=1000  LowerSaturationLimit=0
  Product : Product  RndMeth=Zero
  Product1 : Product  RndMeth=Zero
  Scope : Scope
      settings: SaveName=ScopeData18
  Sum : Sum  Inputs=|++
  Sum1 : Sum  Inputs=|+-
  Vehicle Mass : Gain  Gain=1/m
  Vehicle Mass1 : Gain  Gain=1/m
  Vehicle Moment of Inertial : Gain  Gain=1/Jz
  Longitudinal speed [m/s] : Outport
  Lateral speed [m/s] : Outport  Port=2
  Yaw rate [rad/s] : Outport  Port=3
  wires:
  Integrator2/1 -> Yaw rate [rad/s]/1, Product/2, Product1/2  "r"
  Moment [Nm]/1 -> Vehicle Moment of Inertial/1  "M"
  Integrator1/1 -> Product/1, Lateral speed [m/s]/1  "Vy"
  Integrator3/1 -> Longitudinal speed [m/s]/1, Product1/1, Scope/1  "Vx"
  Vehicle Moment of Inertial/1 -> Integrator2/1
  Vehicle Mass1/1 -> Sum1/1
  Lateral force [N]/1 -> Vehicle Mass1/1  "Fy"
  Vehicle Mass/1 -> Sum/1
  Sum1/1 -> Integrator1/1
  Product1/1 -> Sum1/2
  Sum/1 -> Integrator3/1
  Product/1 -> Sum/2
  Longitudinal force [N]/1 -> Vehicle Mass/1

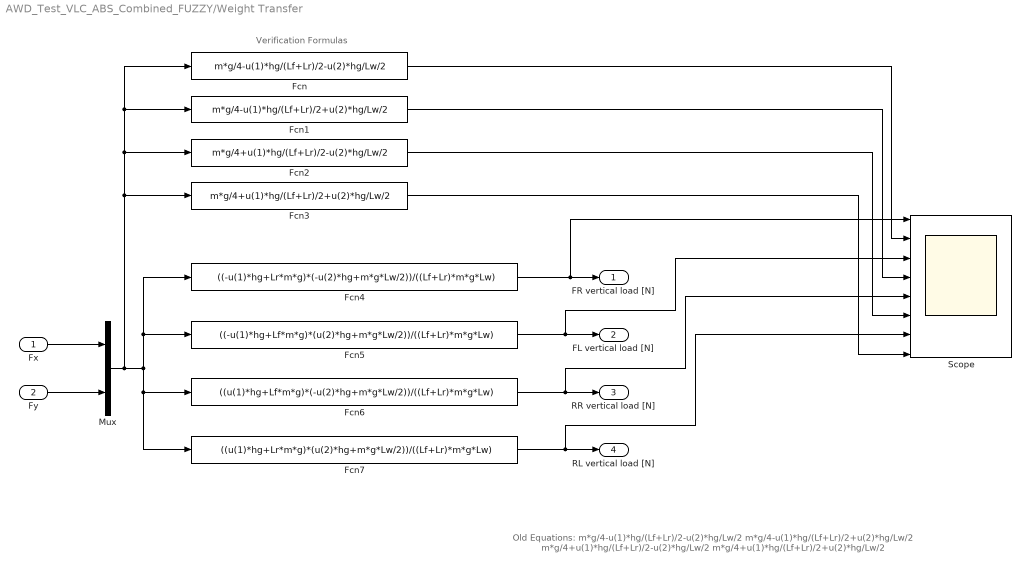
== system AWD_Test_VLC_ABS_Combined_FUZZY/Weight Transfer ==
  note: Old Equations:
      | m*g/4-u(1)*hg/(Lf+Lr)/2-u(2)*hg/Lw/2
      | m*g/4-u(1)*hg/(Lf+Lr)/2+u(2)*hg/Lw/2
      | m*g/4+u(1)*hg/(Lf+Lr)/2-u(2)*hg/Lw/2
      | m*g/4+u(1)*hg/(Lf+Lr)/2+u(2)*hg/Lw/2
  note: Verification Formulas
  Fx : Inport
  Fy : Inport  Port=2
  Fcn : Fcn  Expr=m*g/4-u(1)*hg/(Lf+Lr)/2-u(2)*hg/Lw/2
  Fcn1 : Fcn  Expr=m*g/4-u(1)*hg/(Lf+Lr)/2+u(2)*hg/Lw/2
  Fcn2 : Fcn  Expr=m*g/4+u(1)*hg/(Lf+Lr)/2-u(2)*hg/Lw/2
  Fcn3 : Fcn  Expr=m*g/4+u(1)*hg/(Lf+Lr)/2+u(2)*hg/Lw/2
  Fcn4 : Fcn  Expr=((-u(1)*hg+Lr*m*g)*(-u(2)*hg+m*g*Lw/2))/((Lf+Lr)*m*g*Lw)
  Fcn5 : Fcn  Expr=((-u(1)*hg+Lf*m*g)*(u(2)*hg+m*g*Lw/2))/((Lf+Lr)*m*g*Lw)
  Fcn6 : Fcn  Expr=((u(1)*hg+Lf*m*g)*(-u(2)*hg+m*g*Lw/2))/((Lf+Lr)*m*g*Lw)
  Fcn7 : Fcn  Expr=((u(1)*hg+Lr*m*g)*(u(2)*hg+m*g*Lw/2))/((Lf+Lr)*m*g*Lw)
  Mux : Mux  Inputs=2
  Scope : Scope  NumInputPorts=8
      settings: TimeRange=20  YMin=0~3100~3800~4000~3100~3100~4000~4000  YMax=10000~3400~4400~4300~3400~3400~4300~4300  SaveName=ScopeData6  MaxDataPoints=21000
  FR vertical load [N] : Outport
  FL vertical load [N] : Outport  Port=2
  RR vertical load [N] : Outport  Port=3
  RL vertical load [N] : Outport  Port=4
  wires:
  Fy/1 -> Mux/2
  Fx/1 -> Mux/1
  Fcn4/1 -> FR vertical load [N]/1, Scope/1
  Fcn5/1 -> FL vertical load [N]/1, Scope/3
  Fcn6/1 -> RR vertical load [N]/1, Scope/5
  Fcn7/1 -> RL vertical load [N]/1, Scope/7
  Fcn/1 -> Scope/2
  Fcn1/1 -> Scope/4
  Fcn2/1 -> Scope/6
  Fcn3/1 -> Scope/8
  Mux/1 -> Fcn4/1, Fcn5/1, Fcn6/1, Fcn7/1, Fcn3/1, Fcn2/1, Fcn1/1, Fcn/1

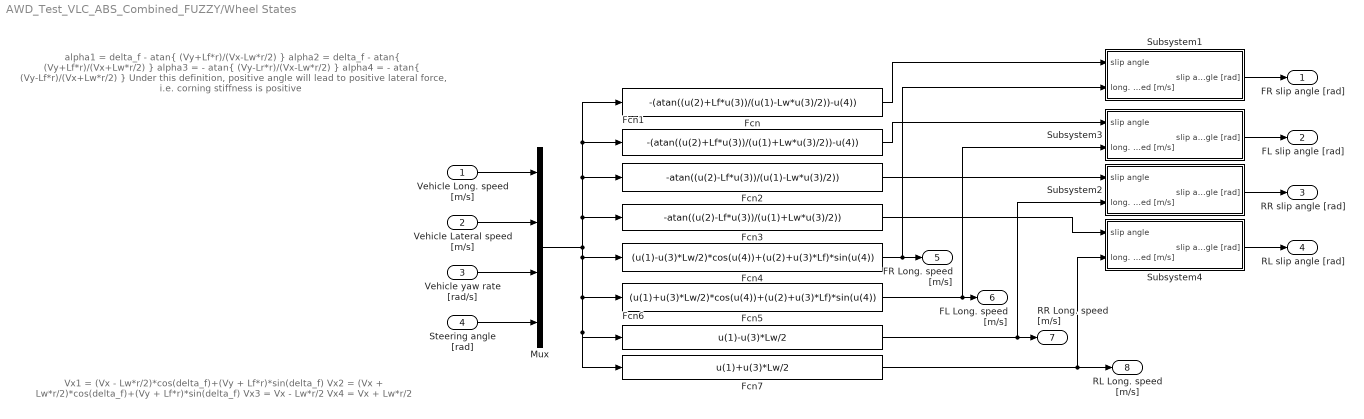
== system AWD_Test_VLC_ABS_Combined_FUZZY/Wheel States ==
  note: alpha1 = delta_f - atan{ (Vy+Lf*r)/(Vx-Lw*r/2) }
      | alpha2 = delta_f - atan{ (Vy+Lf*r)/(Vx+Lw*r/2) }
      | alpha3 = - atan{ (Vy-Lr*r)/(Vx-Lw*r/2) }
      | alpha4 = - atan{ (Vy-Lf*r)/(Vx+Lw*r/2) }
      | Under this definition, positive angle will lead to  positive lateral force,
      | i.e. corning stiffness is positive
  note: Vx1 = (Vx - Lw*r/2)*cos(delta_f)+(Vy + Lf*r)*sin(delta_f)
      | Vx2 = (Vx + Lw*r/2)*cos(delta_f)+(Vy + Lf*r)*sin(delta_f)
      | Vx3 = Vx - Lw*r/2
      | Vx4 = Vx + Lw*r/2
  Vehicle Long. speed [m/s] : Inport
  Vehicle Lateral speed [m/s] : Inport  Port=2
  Vehicle yaw rate [rad/s] : Inport  Port=3
  Steering angle [rad] : Inport  Port=4
  Fcn : Fcn  Expr=-(atan((u(2)+Lf*u(3))/(u(1)-Lw*u(3)/2))-u(4))
  Fcn1 : Fcn  Expr=-(atan((u(2)+Lf*u(3))/(u(1)+Lw*u(3)/2))-u(4))
  Fcn2 : Fcn  Expr=-atan((u(2)-Lf*u(3))/(u(1)-Lw*u(3)/2))
  Fcn3 : Fcn  Expr=-atan((u(2)-Lf*u(3))/(u(1)+Lw*u(3)/2))
  Fcn4 : Fcn  Expr=(u(1)-u(3)*Lw/2)*cos(u(4))+(u(2)+u(3)*Lf)*sin(u(4))
  Fcn5 : Fcn  Expr=(u(1)+u(3)*Lw/2)*cos(u(4))+(u(2)+u(3)*Lf)*sin(u(4))
  Fcn6 : Fcn  Expr=u(1)-u(3)*Lw/2
  Fcn7 : Fcn  Expr=u(1)+u(3)*Lw/2
  Mux : Mux
  Subsystem1 : Subsystem
  Subsystem2 : Subsystem
  Subsystem3 : Subsystem
  Subsystem4 : Subsystem
  "FR slip angle [rad] " : Outport
  "FL slip angle [rad] " : Outport  Port=2
  "RR slip angle [rad] " : Outport  Port=3
  "RL slip angle [rad] " : Outport  Port=4
  FR Long. speed [m/s] : Outport  Port=5
  FL Long. speed [m/s] : Outport  Port=6
  RR Long. speed [m/s] : Outport  Port=7
  RL Long. speed [m/s] : Outport  Port=8
  wires:
  Vehicle yaw rate [rad/s]/1 -> Mux/3
  Vehicle Lateral speed [m/s]/1 -> Mux/2
  Vehicle Long. speed [m/s]/1 -> Mux/1
  Steering angle [rad]/1 -> Mux/4
  Fcn4/1 -> FR Long. speed [m/s]/1, Subsystem1/2(long. speed [m/s])
  Fcn5/1 -> FL Long. speed [m/s]/1, Subsystem3/2(long. speed [m/s])
  Fcn6/1 -> RR Long. speed [m/s]/1, Subsystem2/2(long. speed [m/s])
  Fcn7/1 -> RL Long. speed [m/s]/1, Subsystem4/2(long. speed [m/s])
  Mux/1 -> Fcn5/1, Fcn7/1, Fcn6/1, Fcn4/1, Fcn3/1, Fcn2/1, Fcn1/1, Fcn/1
  Subsystem1/1(slip angle [rad]) -> "FR slip angle [rad] "/1
  Fcn/1 -> Subsystem1/1(slip angle)
  Subsystem3/1(slip angle [rad]) -> "FL slip angle [rad] "/1
  Fcn1/1 -> Subsystem3/1(slip angle)
  Fcn2/1 -> Subsystem2/1(slip angle)
  Fcn3/1 -> Subsystem4/1(slip angle)
  Subsystem2/1(slip angle [rad]) -> "RR slip angle [rad] "/1
  Subsystem4/1(slip angle [rad]) -> "RL slip angle [rad] "/1

== system AWD_Test_VLC_ABS_Combined_FUZZY/ABS/VLC Control/FL Slip Controller ==
  Slip Ratio [%] : Inport
  ABS Fuzzy Controller : fuzblock/Fuzzy Logic  Controller  with Ruleviewer  SystemSampleTime=-1  fismatrix=Fuzzy_Slip_Ctl_ABS  Ts=.1
  Derivative : Derivative
  Mux1 : Mux  Inputs=2
  Scope : Scope
      settings: YMin=1  YMax=1  SaveName=ScopeData8
  Scope1 : Scope
      settings: YMin=1  YMax=1  SaveName=ScopeData17
  VLC Fuzzy Controller : fuzblock/Fuzzy Logic  Controller  with Ruleviewer  SystemSampleTime=-1  fismatrix=Fuzzy_Slip_Ctl_VLC  Ts=.1
  T_lim_Accel : Outport
  T_lim_Brake : Outport  Port=2
  wires:
  Mux1/1 -> VLC Fuzzy Controller/1, ABS Fuzzy Controller/1
  Slip Ratio [%]/1 -> Derivative/1, Mux1/2
  Derivative/1 -> Mux1/1
  VLC Fuzzy Controller/1 -> T_lim_Accel/1, Scope/1
  ABS Fuzzy Controller/1 -> T_lim_Brake/1, Scope1/1

== system AWD_Test_VLC_ABS_Combined_FUZZY/ABS/VLC Control/FR Slip Controller ==
  Slip Ratio [%] : Inport
  ABS Fuzzy Controller : fuzblock/Fuzzy Logic  Controller  with Ruleviewer  SystemSampleTime=-1  fismatrix=Fuzzy_Slip_Ctl_ABS  Ts=.1
  Derivative : Derivative
  Mux1 : Mux  Inputs=2
  Scope : Scope
      settings: SaveName=ScopeData8
  Scope1 : Scope
      settings: SaveName=ScopeData17
  VLC Fuzzy Controller : fuzblock/Fuzzy Logic  Controller  with Ruleviewer  SystemSampleTime=-1  fismatrix=Fuzzy_Slip_Ctl_VLC  Ts=.1
  T_lim_Accel : Outport
  T_lim_Brake : Outport  Port=2
  wires:
  Mux1/1 -> VLC Fuzzy Controller/1, ABS Fuzzy Controller/1
  Slip Ratio [%]/1 -> Derivative/1, Mux1/2
  Derivative/1 -> Mux1/1
  VLC Fuzzy Controller/1 -> T_lim_Accel/1, Scope/1
  ABS Fuzzy Controller/1 -> T_lim_Brake/1, Scope1/1

== system AWD_Test_VLC_ABS_Combined_FUZZY/ABS/VLC Control/RL Slip Controller ==
  Slip Ratio [%] : Inport
  ABS Fuzzy Controller : fuzblock/Fuzzy Logic  Controller  with Ruleviewer  SystemSampleTime=-1  fismatrix=Fuzzy_Slip_Ctl_ABS  Ts=.1
  Derivative : Derivative
  Mux1 : Mux  Inputs=2
  Scope : Scope
      settings: SaveName=ScopeData8
  Scope1 : Scope
      settings: SaveName=ScopeData17
  VLC Fuzzy Controller : fuzblock/Fuzzy Logic  Controller  with Ruleviewer  SystemSampleTime=-1  fismatrix=Fuzzy_Slip_Ctl_VLC  Ts=.1
  T_lim_Accel : Outport
  T_lim_Brake : Outport  Port=2
  wires:
  Mux1/1 -> VLC Fuzzy Controller/1, ABS Fuzzy Controller/1
  Slip Ratio [%]/1 -> Derivative/1, Mux1/2
  Derivative/1 -> Mux1/1
  VLC Fuzzy Controller/1 -> T_lim_Accel/1, Scope/1
  ABS Fuzzy Controller/1 -> T_lim_Brake/1, Scope1/1

== system AWD_Test_VLC_ABS_Combined_FUZZY/ABS/VLC Control/RR Slip Controller ==
  Slip Ratio [%] : Inport
  ABS Fuzzy Controller : fuzblock/Fuzzy Logic  Controller  with Ruleviewer  SystemSampleTime=-1  fismatrix=Fuzzy_Slip_Ctl_ABS  Ts=.1
  Derivative : Derivative
  Mux1 : Mux  Inputs=2
  Scope : Scope
      settings: SaveName=ScopeData8
  Scope1 : Scope
      settings: SaveName=ScopeData17
  VLC Fuzzy Controller : fuzblock/Fuzzy Logic  Controller  with Ruleviewer  SystemSampleTime=-1  fismatrix=Fuzzy_Slip_Ctl_VLC  Ts=.1
  T_lim_Accel : Outport
  T_lim_Brake : Outport  Port=2
  wires:
  Mux1/1 -> VLC Fuzzy Controller/1, ABS Fuzzy Controller/1
  Slip Ratio [%]/1 -> Derivative/1, Mux1/2
  Derivative/1 -> Mux1/1
  VLC Fuzzy Controller/1 -> T_lim_Accel/1, Scope/1
  ABS Fuzzy Controller/1 -> T_lim_Brake/1, Scope1/1

== system AWD_Test_VLC_ABS_Combined_FUZZY/ABS/VLC Control/Yaw Reference/Error Generator ==
  Longitudinal Speed [m/s] : Inport
  lateral speed [m/s] : Inport  Port=2
  yaw rate [rad/s] : Inport  Port=3
  Steering Angle [rad] : Inport  Port=4
  Desired Yaw Calc : Fcn  Expr=(u(1))/(((((Lr+Lf)^(2))*(cos(u(2))/sin(u(2)))^(2))+(Lr)^(2))^(1/2))
  Mux1 : Mux  Inputs=2
  Mux2 : Mux  Inputs=2
  Scope1 : Scope
      settings: YMin=2.125  YMax=2.525  SaveName=ScopeData24
  Scope2 : Scope
      settings: YMin=2.125  YMax=2.525  SaveName=ScopeData25
  Sum : Sum  Inputs=+-|
  Velocity Magnitude : Fcn  Expr=((u(1))^2 + (u(2))^2)^(1/2)
  Yaw Error [rad/s] : Outport
  Steering Angle Out [rad] : Outport  Port=2
  wires:
  Mux1/1 -> Desired Yaw Calc/1
  lateral speed [m/s]/1 -> Mux2/2
  Longitudinal Speed [m/s]/1 -> Mux2/1
  Mux2/1 -> Velocity Magnitude/1
  Velocity Magnitude/1 -> Mux1/1
  Steering Angle [rad]/1 -> Mux1/2, Steering Angle Out [rad]/1
  yaw rate [rad/s]/1 -> Sum/2
  Desired Yaw Calc/1 -> Sum/1, Scope2/1
  Sum/1 -> Yaw Error [rad/s]/1, Scope1/1  "Yaw error"

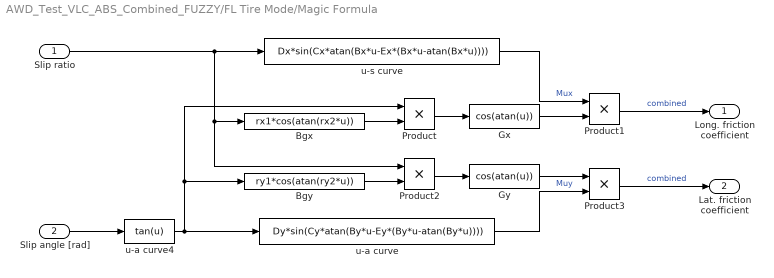
== system AWD_Test_VLC_ABS_Combined_FUZZY/FL Tire Mode/Magic Formula ==
  Slip ratio : Inport
  Slip angle [rad] : Inport  Port=2
  Bgx : Fcn  Expr=rx1*cos(atan(rx2*u))
  Bgy : Fcn  Expr=ry1*cos(atan(ry2*u))
  Gx : Fcn  Expr=cos(atan(u))
  Gy : Fcn  Expr=cos(atan(u))
  Product{,1..3} (4 alike) : Product  RndMeth=Zero
  u-a curve : Fcn  Expr=Dy*sin(Cy*atan(By*u-Ey*(By*u-atan(By*u))))
  u-a curve4 : Fcn  Expr=tan(u)
  u-s curve : Fcn  Expr=Dx*sin(Cx*atan(Bx*u-Ex*(Bx*u-atan(Bx*u))))
  Long. friction coefficient : Outport
  Lat. friction coefficient : Outport  Port=2
  wires:
  Bgx/1 -> Product/2
  Bgy/1 -> Product2/2
  Slip angle [rad]/1 -> u-a curve4/1
  Product3/1 -> Lat. friction coefficient/1  "combined"
  Gy/1 -> Product3/1
  Product2/1 -> Gy/1
  Product1/1 -> Long. friction coefficient/1  "combined"
  Gx/1 -> Product1/2
  Product/1 -> Gx/1
  u-a curve4/1 -> Product/1, Bgy/1, u-a curve/1
  Slip ratio/1 -> Bgx/1, Product2/1, u-s curve/1
  u-a curve/1 -> Product3/2  "Muy"
  u-s curve/1 -> Product1/1  "Mux"

== system AWD_Test_VLC_ABS_Combined_FUZZY/FR Tire Mode/Magic Formula ==
  Slip ratio : Inport
  Slip angle [rad] : Inport  Port=2
  Bgx : Fcn  Expr=rx1*cos(atan(rx2*u))
  Bgy : Fcn  Expr=ry1*cos(atan(ry2*u))
  Gx : Fcn  Expr=cos(atan(u))
  Gy : Fcn  Expr=cos(atan(u))
  Product{,1..3} (4 alike) : Product  RndMeth=Zero
  u-a curve : Fcn  Expr=Dy*sin(Cy*atan(By*u-Ey*(By*u-atan(By*u))))
  u-a curve4 : Fcn  Expr=tan(u)
  u-s curve : Fcn  Expr=Dx*sin(Cx*atan(Bx*u-Ex*(Bx*u-atan(Bx*u))))
  Long. firction coefficient : Outport
  Lat. friction coefficient : Outport  Port=2
  wires:
  u-s curve/1 -> Product1/1  "Mux"
  u-a curve/1 -> Product3/2  "Muy"
  Slip ratio/1 -> u-s curve/1, Product2/1, Bgx/1
  u-a curve4/1 -> u-a curve/1, Bgy/1, Product/1
  Product/1 -> Gx/1
  Gx/1 -> Product1/2
  Product1/1 -> Long. firction coefficient/1  "combined"
  Product2/1 -> Gy/1
  Gy/1 -> Product3/1
  Product3/1 -> Lat. friction coefficient/1  "combined"
  Slip angle [rad]/1 -> u-a curve4/1
  Bgy/1 -> Product2/2
  Bgx/1 -> Product/2

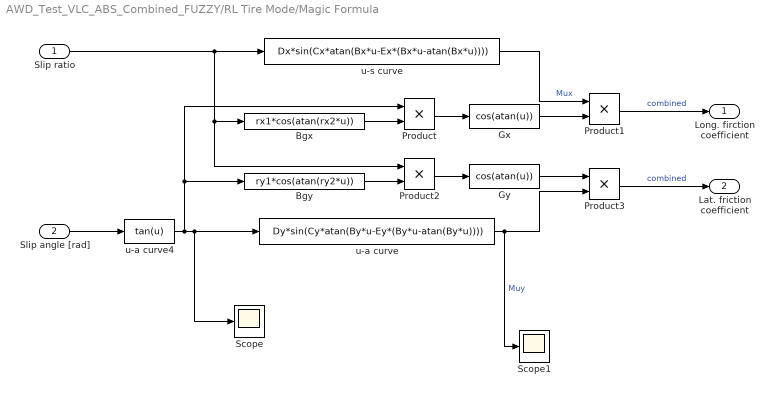
== system AWD_Test_VLC_ABS_Combined_FUZZY/RL Tire Mode/Magic Formula ==
  Slip ratio : Inport
  Slip angle [rad] : Inport  Port=2
  Bgx : Fcn  Expr=rx1*cos(atan(rx2*u))
  Bgy : Fcn  Expr=ry1*cos(atan(ry2*u))
  Gx : Fcn  Expr=cos(atan(u))
  Gy : Fcn  Expr=cos(atan(u))
  Product{,1..3} (4 alike) : Product  RndMeth=Zero
  Scope : Scope
      settings: TimeRange=21
  Scope1 : Scope
      settings: SaveName=ScopeData4
  u-a curve : Fcn  Expr=Dy*sin(Cy*atan(By*u-Ey*(By*u-atan(By*u))))
  u-a curve4 : Fcn  Expr=tan(u)
  u-s curve : Fcn  Expr=Dx*sin(Cx*atan(Bx*u-Ex*(Bx*u-atan(Bx*u))))
  Long. firction coefficient : Outport
  Lat. friction coefficient : Outport  Port=2
  wires:
  Bgx/1 -> Product/2
  Bgy/1 -> Product2/2
  Slip angle [rad]/1 -> u-a curve4/1
  Product3/1 -> Lat. friction coefficient/1  "combined"
  Gy/1 -> Product3/1
  Product2/1 -> Gy/1
  Product1/1 -> Long. firction coefficient/1  "combined"
  Gx/1 -> Product1/2
  Product/1 -> Gx/1
  u-a curve4/1 -> Product/1, Bgy/1, u-a curve/1, Scope/1
  Slip ratio/1 -> Bgx/1, Product2/1, u-s curve/1
  u-a curve/1 -> Product3/2, Scope1/1  "Muy"
  u-s curve/1 -> Product1/1  "Mux"

== system AWD_Test_VLC_ABS_Combined_FUZZY/RR Tire Mode/Magic Formula ==
  Slip ratio : Inport
  Slip angle [rad] : Inport  Port=2
  Bgx : Fcn  Expr=rx1*cos(atan(rx2*u))
  Bgy : Fcn  Expr=ry1*cos(atan(ry2*u))
  Gx : Fcn  Expr=cos(atan(u))
  Gy : Fcn  Expr=cos(atan(u))
  Product{,1..3} (4 alike) : Product  RndMeth=Zero
  u-a curve : Fcn  Expr=Dy*sin(Cy*atan(By*u-Ey*(By*u-atan(By*u))))
  u-a curve4 : Fcn  Expr=tan(u)
  u-s curve : Fcn  Expr=Dx*sin(Cx*atan(Bx*u-Ex*(Bx*u-atan(Bx*u))))
  Long. firction coefficient : Outport
  Lat. friction coefficient : Outport  Port=2
  wires:
  u-s curve/1 -> Product1/1  "Mux"
  u-a curve/1 -> Product3/2  "Muy"
  Slip ratio/1 -> u-s curve/1, Product2/1, Bgx/1
  u-a curve4/1 -> u-a curve/1, Bgy/1, Product/1
  Product/1 -> Gx/1
  Gx/1 -> Product1/2
  Product1/1 -> Long. firction coefficient/1  "combined"
  Product2/1 -> Gy/1
  Gy/1 -> Product3/1
  Product3/1 -> Lat. friction coefficient/1  "combined"
  Slip angle [rad]/1 -> u-a curve4/1
  Bgy/1 -> Product2/2
  Bgx/1 -> Product/2

== system AWD_Test_VLC_ABS_Combined_FUZZY/Wheel States/Subsystem1 ==
  slip angle : Inport
  long. speed [m/s] : Inport  Port=2
  If : If
  Merge1 : Merge
  negative slip angle : Subsystem  TreatAsAtomicUnit=on
  positive slip angle : Subsystem  TreatAsAtomicUnit=on
  slip angle [rad] : Outport
  wires:
  If/2 -> negative slip angle/Action
  negative slip angle/1(-in) -> Merge1/2
  positive slip angle/1(+in) -> Merge1/1
  If/1 -> positive slip angle/Action
  long. speed [m/s]/1 -> If/1
  slip angle/1 -> negative slip angle/1(in), positive slip angle/1(in)
  Merge1/1 -> slip angle [rad]/1

== system AWD_Test_VLC_ABS_Combined_FUZZY/Wheel States/Subsystem2 ==
  slip angle : Inport
  long. speed [m/s] : Inport  Port=2
  If : If
  Merge1 : Merge
  negative slip angle : Subsystem  TreatAsAtomicUnit=on
  positive slip angle : Subsystem  TreatAsAtomicUnit=on
  slip angle [rad] : Outport
  wires:
  Merge1/1 -> slip angle [rad]/1
  slip angle/1 -> positive slip angle/1(in), negative slip angle/1(in)
  long. speed [m/s]/1 -> If/1
  If/1 -> positive slip angle/Action
  positive slip angle/1(+in) -> Merge1/1
  negative slip angle/1(-in) -> Merge1/2
  If/2 -> negative slip angle/Action

== system AWD_Test_VLC_ABS_Combined_FUZZY/Wheel States/Subsystem3 ==
  slip angle : Inport
  long. speed [m/s] : Inport  Port=2
  If : If
  Merge1 : Merge
  negative slip angle : Subsystem  TreatAsAtomicUnit=on
  positive slip angle : Subsystem  TreatAsAtomicUnit=on
  slip angle [rad] : Outport
  wires:
  Merge1/1 -> slip angle [rad]/1
  slip angle/1 -> positive slip angle/1(in), negative slip angle/1(in)
  long. speed [m/s]/1 -> If/1
  If/1 -> positive slip angle/Action
  positive slip angle/1(+in) -> Merge1/1
  negative slip angle/1(-in) -> Merge1/2
  If/2 -> negative slip angle/Action

== system AWD_Test_VLC_ABS_Combined_FUZZY/Wheel States/Subsystem4 ==
  slip angle : Inport
  long. speed [m/s] : Inport  Port=2
  If : If
  Merge1 : Merge
  negative slip angle : Subsystem  TreatAsAtomicUnit=on
  positive slip angle : Subsystem  TreatAsAtomicUnit=on
  slip angle [rad] : Outport
  wires:
  If/2 -> negative slip angle/Action
  negative slip angle/1(-in) -> Merge1/2
  positive slip angle/1(+in) -> Merge1/1
  If/1 -> positive slip angle/Action
  long. speed [m/s]/1 -> If/1
  slip angle/1 -> negative slip angle/1(in), positive slip angle/1(in)
  Merge1/1 -> slip angle [rad]/1

== system AWD_Test_VLC_ABS_Combined_FUZZY/Wheel States/Subsystem1/negative slip angle ==
  in : Inport
  Action Port : ActionPort  ActionType=else
  Gain : Gain  Gain=-1
  -in : Outport
  wires:
  in/1 -> Gain/1
  Gain/1 -> -in/1

== system AWD_Test_VLC_ABS_Combined_FUZZY/Wheel States/Subsystem1/positive slip angle ==
  in : Inport
  Action Port : ActionPort  ActionType=then
  +in : Outport
  wires:
  in/1 -> +in/1

== system AWD_Test_VLC_ABS_Combined_FUZZY/Wheel States/Subsystem2/negative slip angle ==
  in : Inport
  Action Port : ActionPort  ActionType=else
  Gain : Gain  Gain=-1
  -in : Outport
  wires:
  Gain/1 -> -in/1
  in/1 -> Gain/1

== system AWD_Test_VLC_ABS_Combined_FUZZY/Wheel States/Subsystem2/positive slip angle ==
  in : Inport
  Action Port : ActionPort  ActionType=then
  +in : Outport
  wires:
  in/1 -> +in/1

== system AWD_Test_VLC_ABS_Combined_FUZZY/Wheel States/Subsystem3/negative slip angle ==
  in : Inport
  Action Port : ActionPort  ActionType=else
  Gain : Gain  Gain=-1
  -in : Outport
  wires:
  Gain/1 -> -in/1
  in/1 -> Gain/1

== system AWD_Test_VLC_ABS_Combined_FUZZY/Wheel States/Subsystem3/positive slip angle ==
  in : Inport
  Action Port : ActionPort  ActionType=then
  +in : Outport
  wires:
  in/1 -> +in/1

== system AWD_Test_VLC_ABS_Combined_FUZZY/Wheel States/Subsystem4/negative slip angle ==
  in : Inport
  Action Port : ActionPort  ActionType=else
  Gain : Gain  Gain=-1
  -in : Outport
  wires:
  in/1 -> Gain/1
  Gain/1 -> -in/1

== system AWD_Test_VLC_ABS_Combined_FUZZY/Wheel States/Subsystem4/positive slip angle ==
  in : Inport
  Action Port : ActionPort  ActionType=then
  +in : Outport
  wires:
  in/1 -> +in/1
